simulink model "rot1"  (R2015b)
settings: Solver=ode45  StartTime=0.0  StopTime=5  RelTol=1e-3
settings Model: Creator=sebastian  LastModifiedBy=Gabriel
settings DataIOCC: SaveFormat=Array
settings DebuggingCC: SolverPrmCheckMsg=warning
settings HardwareCC: ProdBitPerPointer=32  ProdLargestAtomicFloat=None  ProdIntDivRoundTo=Undefined  ProdEndianess=Unspecified  ProdWordSize=32  ProdHWDeviceType=32-bit Generic
settings GRTTargetCC: GeneratePreprocessorConditionals=Disable all
settings ConfigComp: CovModelRefEnable=Off  CovSFcnEnable=off

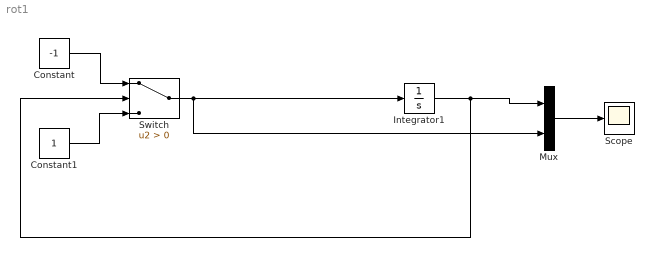
== system rot1 ==
  Constant : Constant  Value=-1
  Constant1 : Constant
  Integrator1 : Integrator  InitialCondition=1
  Mux : Mux  Inputs=2
  Scope : Scope
  Switch : Switch  Criteria=u2 > Threshold  ZeroCross=off
  wires:
  Constant/1 -> Switch/1
  Constant1/1 -> Switch/3
  Mux/1 -> Scope/1
  Integrator1/1 -> Mux/1, Switch/2
  Switch/1 -> Integrator1/1, Mux/2
